simulink model "C28069_LLC_ePWM_V8_230307_PhaeShiftWorking"  (R2022b)
settings: Solver=FixedStepAuto  StartTime=0.0  StopTime=10  RelTol=1e-3  EnableMultiTasking=on
model workspace (MAT data in the model file):
  Comp_DAC = 512
undefined symbols (not defined in the file or in its folder): Down, GPTRIP1SEL, GPTRIP2SEL, PWM_Control, PWM_Gen, PWM_Gen1, SCI_A_Transmit, SCI_A_Transmit_Current_Suffix, SCI_A_Transmit_Duty_Suffix, SCI_A_Transmit_Freq_Suffix, SCI_A_Transmit_OVPFlag_Suffix, SCI_A_Transmit_PFC_Suffix, SCI_A_Transmit_SS_Suffix, SCI_A_Transmit_TBPHS_Suffix, SCI_A_Transmit_VADC_Suffix, SCI_A_Transmit_VAvg_Suffix, SCI_A_Transmit_VBAT_Suffix, SCI_A_Transmit_VBATRef_Suffix, SCI_A_Transmit_Vo_Suffix, TZ1, TZ2, u1, Up
libraries: c2802xlib x92, c280xlib x39, simulink x36, c2000lib x1
(part 17 of 18)

== stateflow chart C28069_LLC_ePWM_V8_230307_PhaeShiftWorking/Softstart @5kHz/GetADC, FaultProtection, SoftStart  @5KHz/SoftStart/If Action Subsystem/SoftStart/Chart1 ==
  note: Under 5KHz, 1 = 0.0002s/cycle
      | 1000 = 0.2s per increment/decrement
  note: [Frequency_Adjusted == Resonant_Frequency]
      | will go here
  note: To initialise the frequency
  (default) -> (junction 47)
  (junction 47) -> (junction 62) [order 2]
  (junction 62) -> (junction 64) : {
      | First_Pass = 1;
      | Soft_Start = 1;
      | Local_counter = 1;
      | SoftStart_OK = 0;
      | }
  (junction 47) -> (junction 48) [order 1] : [PFC_OK]
  (junction 48) -> (junction 49) [order 1] : [First_Pass]
  (junction 48) -> (junction 56) [order 2] : [Soft_Start]
  (junction 56) -> (junction 58) [order 1] : [Local_counter > 400]
      | {
      | Local_counter = 0;
      | }
  (junction 58) -> (junction 74) [order 2]
  (junction 74) -> (junction 81) [order 1] : [[abs(Frequency_Adjusted - Resonant_Frequency)<1]]
  (junction 49) -> (junction 60) : {
      | Frequency_Adjusted = Initial_Frequency;
      | First_Pass = 0;
      | }
  (junction 48) -> (junction 51) [order 3]
  (junction 56) -> (junction 70) [order 2] : {
      | Local_counter = Local_counter +1;
      | }
  (junction 58) -> (junction 68) [order 1] : [Frequency_Adjusted > Resonant_Frequency]
      | {
      | Frequency_Adjusted = Frequency_Adjusted - 0.1;
      | }
  (junction 74) -> (junction 76) [order 2] : [Frequency_Adjusted < Resonant_Frequency]
      |
      | {
      | Frequency_Adjusted = Frequency_Adjusted + 0.1;
      | }
  (junction 81) -> (junction 84) : {
      | SoftStart_OK = 1;
      | Soft_Start = 0;
      | %Frequency_Adjusted = Initial_Frequency;
      | }
  (junction 64) -> (junction 60)
  (junction 60) -> (junction 51)
  (junction 51) -> (junction 70)
  (junction 70) -> (junction 68)
  (junction 68) -> (junction 76)
  (junction 84) -> (junction 76)
  data: SoftStart_OK output; PFC_OK input; Initial_Frequency input; Resonant_Frequency input; Local_counter local =1; Frequency_Adjusted output; First_Pass local =1; Soft_Start local =1

== stateflow chart C28069_LLC_ePWM_V8_230307_PhaeShiftWorking/Softstart @5kHz/GetADC, FaultProtection, SoftStart  @5KHz/SoftStart1/If Action Subsystem/ReservseSoftStart1/Chart1 ==
  note: Under 5KHz, 1 = 0.0002s/cycle
      | 1000 = 0.2s per increment/decrement
  note: [Frequency_Adjusted == Resonant_Frequency]
      | will go here
  note: To initialise the frequency
  note: For increment of 110 (+-5% each DC)
      | Duty_Adjusted @ 660 = 15% Duty
      | '' @ 770 = 10% Duty
      | - - - - - - - - - - - - - - - -
      | 715 + 55 = 15% DutyCycle
      | 660 + 55 (+-2.5%DC) = ~18% DutyCycle = 1us (Minimum required)
  (default) -> (junction 47)
  (junction 47) -> (junction 62) [order 2]
  (junction 62) -> (junction 64) : {
      | First_Pass = 1;
      | Soft_Start = 1;
      | Local_counter = 1;
      | SoftStart_OK = 0;
      | Duty_Adjusted = 100;
      | }
  (junction 47) -> (junction 48) [order 1] : [PFC_OK]
  (junction 48) -> (junction 49) [order 1] : [First_Pass]
  (junction 48) -> (junction 56) [order 2] : [Soft_Start]
  (junction 56) -> (junction 58) [order 1] : [Local_counter > 600]
      | {
      | Local_counter = 0;
      | }
  (junction 58) -> (junction 74) [order 2]
  (junction 74) -> (junction 81) [order 1] : [abs(Frequency_Adjusted - Resonant_Frequency)<1]
  (junction 48) -> (junction 105) [order 4]
  (junction 49) -> (junction 60) : {
      | Frequency_Adjusted = Initial_Frequency;
      | First_Pass = 0;
      | }
  (junction 48) -> (junction 102) [order 3] : [Duty_Adjusted <= 550]
  (junction 56) -> (junction 70) [order 2] : {
      | Local_counter = Local_counter +1;
      | }
  (junction 58) -> (junction 68) [order 1] : [Frequency_Adjusted > Resonant_Frequency]
      | {
      | Frequency_Adjusted = Frequency_Adjusted - 0.1;
      | }
  (junction 74) -> (junction 76) [order 2] : [Frequency_Adjusted < Resonant_Frequency]
      |
      | {
      | Frequency_Adjusted = Frequency_Adjusted + 0.1;
      | }
  (junction 81) -> (junction 84) : {
      | SoftStart_OK = 1;
      | Soft_Start = 0;
      | %%Frequency_Adjusted = Initial_Frequency;
      | }
  (junction 102) -> (junction 105) [order 2] : {
      | Local_counter = Local_counter +1;
      | }
  (junction 105) -> (junction 51)
  (junction 102) -> (junction 108) [order 1] : [Local_counter >600]
      | {
      | Local_counter = 0;
      | }
  (junction 108) -> (junction 51) : {
      | Duty_Adjusted = Duty_Adjusted + 55;
      | }
  (junction 64) -> (junction 60)
  (junction 60) -> (junction 51)
  (junction 51) -> (junction 70)
  (junction 70) -> (junction 68)
  (junction 68) -> (junction 76)
  (junction 84) -> (junction 76)
  data: SoftStart_OK output; Duty_Adjusted output =100; PFC_OK input; Initial_Frequency input; Resonant_Frequency input; Local_counter local =1; Frequency_Adjusted output double; First_Pass local =1; Soft_Start local =1

== stateflow chart C28069_LLC_ePWM_V8_230307_PhaeShiftWorking/Softstart @5kHz/GetADC, FaultProtection, SoftStart  @5KHz/SoftStart1/If Action Subsystem/SoftStart1/Chart ==
  note: Verror = Vbulk_Ref_ADC_adjusted - Vbulk_ADC;
  note: Local variables
      | VbusRefTemp
      | SoftStartCnt
  (default) -> (junction 47)
  (junction 47) -> (junction 50) [order 2]
  (junction 50) -> (junction 52) : {
      | %First_Pass=1;
      | %Soft_Start=1;
      | %SoftStartCnt=1;
      | %Debug=1;
      | }
  (junction 47) -> (junction 5) [order 1] : [PFC_OK]
  (junction 5) -> (junction 7) [order 1] : [First_Pass]
  (junction 5) -> (junction 15) [order 2] : [Soft_Start]
  (junction 15) -> (junction 18) [order 1] : [SoftStartCnt>15]
      | %% 1 count = 0.2ms (5kHz)
      | %% 10 counts = 2ms
  (junction 18) -> (junction 23) [order 2] : %{Debug=Vbulk_Ref_ADC_adjusted;}
  (junction 23) -> (junction 31) : %{Debug=6;}
  (junction 31) -> (junction 55) [order 1] : [abs(VBAT_Ref_adjusted - VBAT_Ref)<0.9]
  (junction 7) -> (junction 10) : {
      | VBAT_Ref_adjusted = VBAT_Value/30;
      | %Vbulk_Ref_ADC_adjusted = Vbulk_Ref_ADC;
      | First_Pass = 0;
      | %Debug=2;
      |
      | }
  (junction 5) -> (junction 38) [order 3] : {
      | SoftStart_OK = 1;
      | %Debug=3;
      | %Vbulk_Ref_ADC_adjusted=Vbulk_Ref_ADC;
      | }
  (junction 15) -> (junction 20) [order 2] : {
      | SoftStartCnt = SoftStartCnt + 1;
      | %Debug=4;
      | }
      | %% incerase the counter first.
  (junction 18) -> (junction 64) [order 1] : [VBAT_Ref_adjusted < VBAT_Ref]
      | {VBAT_Ref_adjusted = VBAT_Ref_adjusted + 0.1;}
      | %% Increase the reference voltage
  (junction 23) -> (junction 26) [commented out] : [VBAT_Ref_adjusted > VBAT_Ref]
      | {VBAT_Ref_adjusted = VBAT_Ref_adjusted - 0.1;
      | }
      | %% Reduce the reference voltage
  (junction 31) -> (junction 33) [order 2] : {
      | Soft_Start=0;
      | SoftStartCnt=0;
      | %Debug=7;
      | VBAT_Ref_adjusted=VBAT_Ref;
      | }
      | %% End soft start
  (junction 55) -> (junction 57) : {
      | Soft_Start=0;
      | SoftStartCnt=0;
      | VBAT_Ref_adjusted=VBAT_Ref;
      | %Debug=8;
      | }
  (junction 64) -> (junction 28) [order 2]
  (junction 64) -> (junction 28) [order 1] : [VBAT_Ref_adjusted < (VBAT_Value/30)]
      | {VBAT_Ref_adjusted = (VBAT_Value/30) ;}
      | %% Increase the reference voltage
  (junction 52) -> (junction 10)
  (junction 10) -> (junction 38)
  (junction 26) -> (junction 28)
  (junction 33) -> (junction 26)
  (junction 57) -> (junction 33)
  (junction 20) -> (junction 38)
  (junction 28) -> (junction 20)
  data: PFC_OK input; VBAT_Value input; VbusRefTemp local =0; SoftStartCnt local =0; VBAT_Ref input double; VBAT_Ref_adjusted output double =0; Vbulk_Ref_ADC_Hard_Value local =0; First_Pass1 local; First_Pass local =1; Soft_Start local =1; SoftStart_OK output

== stateflow chart C28069_LLC_ePWM_V8_230307_PhaeShiftWorking/Softstart @5kHz/GetADC, FaultProtection, SoftStart  @5KHz/SoftStart1/If Action Subsystem/SoftStart1/Chart1 ==
  note: Under 5KHz, 1 = 0.0002s/cycle
      | 1000 = 0.2s per increment/decrement
  note: [Frequency_Adjusted == Resonant_Frequency]
      | will go here
  note: To initialise the frequency
  (default) -> (junction 47)
  (junction 47) -> (junction 62) [order 2]
  (junction 62) -> (junction 64) : {
      | First_Pass = 1;
      | Soft_Start = 1;
      | Local_counter = 1;
      | SoftStart_OK = 0;
      | }
  (junction 47) -> (junction 48) [order 1] : [PFC_OK]
  (junction 48) -> (junction 49) [order 1] : [First_Pass]
  (junction 48) -> (junction 56) [order 2] : [Soft_Start]
  (junction 56) -> (junction 58) [order 1] : [Local_counter > 400]
      | {
      | Local_counter = 0;
      | }
  (junction 58) -> (junction 74) [order 2]
  (junction 74) -> (junction 81) [order 1] : [[abs(Frequency_Adjusted - Resonant_Frequency)<1]]
  (junction 49) -> (junction 60) : {
      | Frequency_Adjusted = Initial_Frequency;
      | First_Pass = 0;
      | }
  (junction 48) -> (junction 51) [order 3]
  (junction 56) -> (junction 70) [order 2] : {
      | Local_counter = Local_counter +1;
      | }
  (junction 58) -> (junction 68) [order 1] : [Frequency_Adjusted > Resonant_Frequency]
      | {
      | Frequency_Adjusted = Frequency_Adjusted - 0.1;
      | }
  (junction 74) -> (junction 76) [order 2] : [Frequency_Adjusted < Resonant_Frequency]
      |
      | {
      | Frequency_Adjusted = Frequency_Adjusted + 0.1;
      | }
  (junction 81) -> (junction 84) : {
      | SoftStart_OK = 1;
      | Soft_Start = 0;
      | %Frequency_Adjusted = Initial_Frequency;
      | }
  (junction 64) -> (junction 60)
  (junction 60) -> (junction 51)
  (junction 51) -> (junction 70)
  (junction 70) -> (junction 68)
  (junction 68) -> (junction 76)
  (junction 84) -> (junction 76)
  data: SoftStart_OK output; PFC_OK input; Initial_Frequency input; Resonant_Frequency input; Local_counter local =1; Frequency_Adjusted output; First_Pass local =1; Soft_Start local =1

== stateflow chart C28069_LLC_ePWM_V8_230307_PhaeShiftWorking/Softstart @5kHz/GetADC, FaultProtection, SoftStart  @5KHz/SoftStart1/ReservseSoftStart/Chart1 ==
  note: Under 5KHz, 1 = 0.0002s/cycle
      | 1000 = 0.2s per increment/decrement
  note: [Frequency_Adjusted == Resonant_Frequency]
      | will go here
  note: To initialise the frequency
  note: For increment of 110 (+-5% each DC)
      | Duty_Adjusted @ 660 = 15% Duty
      | '' @ 770 = 10% Duty
      | - - - - - - - - - - - - - - - -
      | 715 + 55 = 15% DutyCycle
      | 660 + 55 (+-2.5%DC) = ~18% DutyCycle = 1us (Minimum required)
  (default) -> (junction 47)
  (junction 47) -> (junction 62) [order 2]
  (junction 62) -> (junction 64) : {
      | First_Pass = 1;
      | Soft_Start = 1;
      | Local_counter = 1;
      | SoftStart_OK = 0;
      | Duty_Adjusted = 100;
      | }
  (junction 47) -> (junction 48) [order 1] : [PFC_OK]
  (junction 48) -> (junction 49) [order 1] : [First_Pass]
  (junction 48) -> (junction 56) [order 2] : [Soft_Start]
  (junction 56) -> (junction 58) [order 1] : [Local_counter > 600]
      | {
      | Local_counter = 0;
      | }
  (junction 58) -> (junction 74) [order 2]
  (junction 74) -> (junction 81) [order 1] : [abs(Frequency_Adjusted - Resonant_Frequency)<1]
  (junction 48) -> (junction 105) [order 4]
  (junction 49) -> (junction 60) : {
      | Frequency_Adjusted = Initial_Frequency;
      | First_Pass = 0;
      | }
  (junction 48) -> (junction 102) [order 3] : [Duty_Adjusted <= 550]
  (junction 56) -> (junction 70) [order 2] : {
      | Local_counter = Local_counter +1;
      | }
  (junction 58) -> (junction 68) [order 1] : [Frequency_Adjusted > Resonant_Frequency]
      | {
      | Frequency_Adjusted = Frequency_Adjusted - 0.1;
      | }
  (junction 74) -> (junction 76) [order 2] : [Frequency_Adjusted < Resonant_Frequency]
      |
      | {
      | Frequency_Adjusted = Frequency_Adjusted + 0.1;
      | }
  (junction 81) -> (junction 84) : {
      | SoftStart_OK = 1;
      | Soft_Start = 0;
      | %%Frequency_Adjusted = Initial_Frequency;
      | }
  (junction 102) -> (junction 105) [order 2] : {
      | Local_counter = Local_counter +1;
      | }
  (junction 105) -> (junction 51)
  (junction 102) -> (junction 108) [order 1] : [Local_counter >600]
      | {
      | Local_counter = 0;
      | }
  (junction 108) -> (junction 51) : {
      | Duty_Adjusted = Duty_Adjusted + 55;
      | }
  (junction 64) -> (junction 60)
  (junction 60) -> (junction 51)
  (junction 51) -> (junction 70)
  (junction 70) -> (junction 68)
  (junction 68) -> (junction 76)
  (junction 84) -> (junction 76)
  data: SoftStart_OK output; Duty_Adjusted output =100; PFC_OK input; Initial_Frequency input; Resonant_Frequency input; Local_counter local =1; Frequency_Adjusted output double; First_Pass local =1; Soft_Start local =1

== stateflow chart C28069_LLC_ePWM_V8_230307_PhaeShiftWorking/GetADC, FaultProtection, SoftStart  @5KHz/Counter with reset Min output = 1 Max output = Counter reset value ==
  (default) -> (junction 1)
  (junction 1) -> (junction 17) [order 2]
  (junction 1) -> (junction 3) [order 1]
  (junction 17) -> (junction 19) : [(Counter==Number_of_counts) & Latch_switch]
      | {Counter=Number_of_counts;}
  (junction 1) -> (junction 7) [order 3] : {Counter = Counter + 1;}
  (junction 3) -> (junction 5) : [(Counter==Number_of_counts+1) & (~Latch_switch)]
      | {Counter=1;}
  (junction 19) -> (junction 7)
  (junction 5) -> (junction 7)
  data: Number_of_counts input; Counter output double =0; Latch_switch input

== stateflow chart C28069_LLC_ePWM_V8_230307_PhaeShiftWorking/Softstart @5kHz/GetADC, FaultProtection, SoftStart  @5KHz/SoftStart1/SoftStart/Chart ==
  note: Verror = Vbulk_Ref_ADC_adjusted - Vbulk_ADC;
  note: Local variables
      | VbusRefTemp
      | SoftStartCnt
  (default) -> (junction 47)
  (junction 47) -> (junction 50) [order 2]
  (junction 50) -> (junction 52) : {
      | First_Pass=1;
      | Soft_Start=1;
      | SoftStartCnt=1;
      | %Debug=1;
      | }
  (junction 47) -> (junction 5) [order 1] : [PFC_OK]
  (junction 5) -> (junction 7) [order 1] : [First_Pass]
  (junction 5) -> (junction 15) [order 2] : [Soft_Start]
  (junction 15) -> (junction 18) [order 1] : [SoftStartCnt>100]
      | %% At every 5 cycles (total 1ms),
  (junction 18) -> (junction 23) [order 2] : %{Debug=Vbulk_Ref_ADC_adjusted;}
  (junction 23) -> (junction 31) [order 2] : %{Debug=6;}
  (junction 31) -> (junction 55) [order 1] : [abs(VBAT_Ref_adjusted - VBAT_Ref)<1]
  (junction 7) -> (junction 10) : {
      | VBAT_Ref_adjusted = VBAT_Value;
      | %Vbulk_Ref_ADC_adjusted = Vbulk_Ref_ADC;
      | First_Pass = 0;
      | %Debug=2;
      |
      | }
  (junction 5) -> (junction 38) [order 3] : {
      | %Debug=3;
      | %Vbulk_Ref_ADC_adjusted=Vbulk_Ref_ADC;
      | }
  (junction 15) -> (junction 20) [order 2] : {
      | SoftStartCnt = SoftStartCnt + 1;
      | %Debug=4;
      | }
      | %% incerase the counter first.
  (junction 18) -> (junction 64) [order 1] : [VBAT_Ref_adjusted < VBAT_Ref]
      | {VBAT_Ref_adjusted = VBAT_Ref_adjusted + 0.1;}
      | %% Increase the reference voltage
  (junction 23) -> (junction 26) [order 1] : [VBAT_Ref_adjusted > VBAT_Ref]
      | {VBAT_Ref_adjusted = VBAT_Ref_adjusted - 0.1;
      | }
      | %% Reduce the reference voltage
  (junction 31) -> (junction 33) [order 2] : {
      | Soft_Start=0;
      | SoftStartCnt=0;
      | %Debug=7;
      | }
      | %% End soft start
  (junction 55) -> (junction 57) : {
      | Soft_Start=0;
      | SoftStartCnt=0;
      | VBAT_Ref_adjusted=VBAT_Ref;
      | %Debug=8;
      | }
  (junction 64) -> (junction 28) [order 2]
  (junction 64) -> (junction 28) [order 1] : [VBAT_Ref_adjusted < VBAT_Value]
      | {VBAT_Ref_adjusted = VBAT_Value ;}
      | %% Increase the reference voltage
  (junction 52) -> (junction 10)
  (junction 10) -> (junction 38)
  (junction 26) -> (junction 28)
  (junction 33) -> (junction 26)
  (junction 57) -> (junction 33)
  (junction 20) -> (junction 38)
  (junction 28) -> (junction 20)
  data: PFC_OK input; VBAT_Value input; VbusRefTemp local =0; SoftStartCnt local =0; VBAT_Ref input double; VBAT_Ref_adjusted output double =0; Vbulk_Ref_ADC_Hard_Value local =0; First_Pass1 local; First_Pass local =1; Soft_Start local =1

== stateflow chart C28069_LLC_ePWM_V8_230307_PhaeShiftWorking/Softstart @5kHz/GetADC, FaultProtection, SoftStart  @5KHz/SoftStart1/SoftStart/Chart1 ==
  note: Under 5KHz, 1 = 0.0002s/cycle
      | 1000 = 0.2s per increment/decrement
  note: [Frequency_Adjusted == Resonant_Frequency]
      | will go here
  note: To initialise the frequency
  (default) -> (junction 47)
  (junction 47) -> (junction 62) [order 2]
  (junction 62) -> (junction 64) : {
      | First_Pass = 1;
      | Soft_Start = 1;
      | Local_counter = 1;
      | SoftStart_OK = 0;
      | }
  (junction 47) -> (junction 48) [order 1] : [PFC_OK]
  (junction 48) -> (junction 49) [order 1] : [First_Pass]
  (junction 48) -> (junction 56) [order 2] : [Soft_Start]
  (junction 56) -> (junction 58) [order 1] : [Local_counter > 400]
      | {
      | Local_counter = 0;
      | }
  (junction 58) -> (junction 74) [order 2]
  (junction 74) -> (junction 81) [order 1] : [[abs(Frequency_Adjusted - Resonant_Frequency)<1]]
  (junction 49) -> (junction 60) : {
      | Frequency_Adjusted = Initial_Frequency;
      | First_Pass = 0;
      | }
  (junction 48) -> (junction 51) [order 3]
  (junction 56) -> (junction 70) [order 2] : {
      | Local_counter = Local_counter +1;
      | }
  (junction 58) -> (junction 68) [order 1] : [Frequency_Adjusted > Resonant_Frequency]
      | {
      | Frequency_Adjusted = Frequency_Adjusted - 0.1;
      | }
  (junction 74) -> (junction 76) [order 2] : [Frequency_Adjusted < Resonant_Frequency]
      |
      | {
      | Frequency_Adjusted = Frequency_Adjusted + 0.1;
      | }
  (junction 81) -> (junction 84) : {
      | SoftStart_OK = 1;
      | Soft_Start = 0;
      | %Frequency_Adjusted = Initial_Frequency;
      | }
  (junction 64) -> (junction 60)
  (junction 60) -> (junction 51)
  (junction 51) -> (junction 70)
  (junction 70) -> (junction 68)
  (junction 68) -> (junction 76)
  (junction 84) -> (junction 76)
  data: SoftStart_OK output; PFC_OK input; Initial_Frequency input; Resonant_Frequency input; Local_counter local =1; Frequency_Adjusted output; First_Pass local =1; Soft_Start local =1

== stateflow chart C28069_LLC_ePWM_V8_230307_PhaeShiftWorking/Softstart @5kHz/GetADC, FaultProtection, SoftStart  @5KHz/UpdatePWM/Close Loop Regulation/If Action Subsystem/Chart ==
  note: Note
      | Voltage drop = Freq increase
  note: When Actual voltage is higher
  note: When Actual voltage is lower
  (default) -> (junction 1)
  (junction 1) -> (junction 16) [order 1] : [input_u>0]{output_y=prev_freq-0.01;}
  (junction 1) -> (junction 17) [order 2] : {output_y=prev_freq+0.01;}
  (junction 16) -> (junction 19) [order 1] : [output_y<100]{output_y=100;}
  (junction 17) -> (junction 19) [order 1] : [output_y>180]{output_y=180;}
  (junction 17) -> (junction 32) [order 2]
  (junction 16) -> (junction 34) [order 2]
  (junction 32) -> (junction 19)
  (junction 34) -> (junction 19)
  (junction 19) -> (junction 22)
  data: output_y output double; input_u input double; prev_freq input double

== stateflow chart C28069_LLC_ePWM_V8_230307_PhaeShiftWorking/CloseLoop & Update @ ADCINT, 50kHz/Close Loop Regulation1/If Action Subsystem/Chart1 ==
  note: [output_freq>180]
      | {
      | output_freq=180;
      | output_deadband =  output_deadband + 1;
      | }
  (default) -> (junction 221)
  (junction 221) -> (junction 223) : {
      | %%y(k) = b0*e(k) + b1*e(k-1) - a1*y(k-1)
      | output_freq = (b0*error) + (b1*error_z1) - (a1*output_z1);
      | }
  (junction 223) -> (junction 239) [order 2] : [output_freq<0.65]
  (junction 223) -> (junction 243) [order 3]
  (junction 239) -> (junction 241) : {output_freq=0.65;}
  (junction 223) -> (junction 225) [order 1] : [output_freq>1.5]
  (junction 243) -> (junction 245)
  (junction 225) -> (junction 237) : {output_freq=1.5;}
  (junction 241) -> (junction 237)
  (junction 245) -> (junction 237)
  (junction 237) -> (junction 233) : {
      | output_z1 = output_freq;
      | error_z1 = error;
      | }
  data: output_freq output double =0; error input double; prev_freq input double; b0 input; b1 input; a1 input; error_z1 local =0; output_z1 local =0

== matlab function C28069_LLC_ePWM_V8_230307_PhaeShiftWorking/UART Reporting @ 1Hz/SCI_A_Transmit_function2/MATLAB Function ==
  data: Main_number input; Digit_5 output; Divider input; Digit_4 output; Digit_3 output; Digit_2 output; Digit_1 output
function [Digit_5,Digit_4,Digit_3,Digit_2,Digit_1]  = fcn(Main_number,Divider)

R_Digit_5 = rem(Main_number,Divider);
Q_Digit_5 = (Main_number-R_Digit_5)/Divider;
Digit_5 = uint8(Q_Digit_5);
%Digit_5 done

R_Digit_4 = rem(R_Digit_5,Divider/10);
Q_Digit_4 = (R_Digit_5-R_Digit_4)/(Divider/10);
Digit_4 = uint8(Q_Digit_4);
%Digit_4 done

R_Digit_3 = rem(R_Digit_4,Divider/100);
Q_Digit_3 = (R_Digit_4-R_Digit_3)/(Divider/100);
Digit_3 = uint8(Q_Digit_3);
%Digit_3 done

R_Digit_2 = rem(R_Digit_3,Divider/1000);
Q_Digit_2 = (R_Digit_3-R_Digit_2)/(Divider/1000);
Digit_2 = uint8(Q_Digit_2);
%Digit_2 done

R_Digit_1 = rem(R_Digit_2,Divider/10000);
Q_Digit_1 = (R_Digit_2-R_Digit_1)/(Divider/10000);
Digit_1 = uint8(Q_Digit_1);
%Digit_1 done
end

== stateflow chart C28069_LLC_ePWM_V8_230307_PhaeShiftWorking/CloseLoop & Update @ ADCINT, 50kHz/Close Loop Regulation1/If Action Subsystem/Chart2 ==
  note: Note
      | Voltage drop = Freq increase
  note: When Actual voltage is higher
  note: When Actual voltage is lower
  note: Note
      | Voltage drop = Freq increase
  note: When Actual voltage is lower
  note: When Actual voltage is higher
  note: If <25V & <47% & freq is 180K
  note: Minor delay of 1KHz,
      | 1 count = 1ms
      | 100 = 100ms delay
  note: Increase Duty
  note: Reduce Duty
  (default) -> (junction 1)
  (junction 17) -> (junction 145) [order 2]
  (junction 1) -> (junction 17) [order 2] : {output_freq=prev_freq+0.05;}
  (junction 1) -> (junction 157) [order 1] : [error>0]
  (junction 157) -> (junction 184) [order 2]
  (junction 184) -> (junction 164) [order 2]
  (junction 145) -> (junction 152)
  (junction 17) -> (junction 141) [order 1] : [output_freq>180]
      | {
      | output_freq=180;
      | output_deadband =  output_deadband + 1;
      | }
  (junction 157) -> (junction 181) [order 1] : [output_deadband>1]
      | {output_deadband = output_deadband - 1;}
  (junction 184) -> (junction 187) [order 1] : [output_freq==0]
      | {output_freq=180;}
  (junction 164) -> (junction 166) : {output_freq=output_freq-0.05;}
  (junction 166) -> (junction 177) [order 2]
  (junction 166) -> (junction 171) [order 1] : [output_freq<100]{output_freq=100;}
  (junction 177) -> (junction 175)
  (junction 141) -> (junction 152) [order 2]
  (junction 152) -> (junction 147)
  (junction 141) -> (junction 143) [order 1] : [output_deadband > 660]
      | {
      | output_deadband = 660;
      | output_freq=0;
      | }
  (junction 147) -> (junction 143)
  (junction 143) -> (junction 181)
  (junction 187) -> (junction 181)
  (junction 171) -> (junction 187)
  (junction 175) -> (junction 171)
  (default) -> (junction 94) [commented out]
  (junction 94) -> (junction 101) [commented out] : {output_freq=prev_freq+0.05;}
  (junction 94) -> (junction 89) [commented out] : [error>0]{output_freq=prev_freq-0.05;}
  (junction 101) -> (junction 98) [commented out] : [output_freq>180]
      | {
      | output_freq=180;
      | %limit_cap = limit_cap + 1;
      | }
  (junction 94) -> (junction 96) [commented out] : [input_u> 0 & duty_output > 56 & prev_freq ==180]
  (junction 89) -> (junction 108) [commented out]
  (junction 101) -> (junction 103) [commented out]
  (junction 89) -> (junction 108) [commented out] : [output_freq<100]{output_freq=100;}
  (junction 98) -> (junction 105) [commented out] : [input_u<0]
  (junction 98) -> (junction 97) [commented out]
  (junction 96) -> (junction 132) [commented out] : {
      | duty_output = duty_output - 55;
      | }
  (junction 105) -> (junction 113) [commented out] : %Need to send CMPA 0 not duty
      | %{duty_output = 0;}
  (junction 105) -> (junction 99) [commented out] : [duty_output <= 660]
  (junction 97) -> (junction 134) [commented out] : %{limit_cap = 0;}
  (junction 99) -> (junction 90) [commented out]
  (junction 99) -> (junction 100) [commented out] : [Local_counter > 600]
      | {
      | Local_counter = 0;
      | }
  (junction 90) -> (junction 113) [commented out] : {Local_counter = Local_counter + 1;}
  (junction 100) -> (junction 117) [commented out] : {
      | duty_output = duty_output + 55;
      | }
  (junction 103) -> (junction 107) [commented out]
  (junction 107) -> (junction 113) [commented out]
  (junction 113) -> (junction 117) [commented out]
  (junction 134) -> (junction 117) [commented out]
  (junction 132) -> (junction 134) [commented out]
  (junction 108) -> (junction 132) [commented out]
  (junction 117) -> (junction 110) [commented out]
  data: output_freq output double; error input double; prev_freq input double; limit_cap local double =0; Local_counter local =0; output_deadband output

== stateflow chart C28069_LLC_ePWM_V8_230307_PhaeShiftWorking/CloseLoop & Update @ ADCINT, 50kHz/Close Loop Regulation1/If Action Subsystem/Chart3 ==
  note: [output_freq>180]
      | {
      | output_freq=180;
      | output_deadband =  output_deadband + 1;
      | }
  (default) -> (junction 221)
  (junction 221) -> (junction 223) : {
      | %%y(k) = b0*e(k) + b1*e(k-1) - a1*y(k-1)
      | output_freq = (b0*error) + (b1*error_z1) - (a1*output_z1);
      | }
  (junction 223) -> (junction 239) [order 2] : [output_freq<0.65]
  (junction 223) -> (junction 243) [order 3]
  (junction 239) -> (junction 241) : {output_freq=0.65;}
  (junction 223) -> (junction 225) [order 1] : [output_freq>1.5]
  (junction 243) -> (junction 245)
  (junction 225) -> (junction 237) : {output_freq=1.5;}
  (junction 241) -> (junction 237)
  (junction 245) -> (junction 237)
  (junction 237) -> (junction 233) : {
      | output_z1 = output_freq;
      | error_z1 = error;
      | }
  data: output_freq output double =0; error input double; prev_freq input double; b0 input; b1 input; a1 input; error_z1 local =0; output_z1 local =0

== stateflow chart C28069_LLC_ePWM_V8_230307_PhaeShiftWorking/GetADC, FaultProtection, SoftStart  @5KHz/UpdatePWM1/Close Loop Regulation/If Action Subsystem/Chart1 ==
  note: [output_freq>180]
      | {
      | output_freq=180;
      | output_deadband =  output_deadband + 1;
      | }
  (default) -> (junction 221)
  (junction 221) -> (junction 223) : {
      | %%y(k) = b0*e(k) + b1*e(k-1) - a1*y(k-1)
      | output_freq = (b0*error) + (b1*error_z1) - (a1*output_z1);
      | }
  (junction 223) -> (junction 239) [order 2] : [output_freq<0.9]
  (junction 223) -> (junction 243) [order 3]
  (junction 239) -> (junction 241) : {output_freq=0.9;}
  (junction 223) -> (junction 225) [order 1] : [output_freq>1.5]
  (junction 243) -> (junction 245)
  (junction 225) -> (junction 237) : {output_freq=1.5;}
  (junction 241) -> (junction 237)
  (junction 245) -> (junction 237)
  (junction 237) -> (junction 233) : {
      | output_z1 = output_freq;
      | error_z1 = error;
      | }
  data: output_freq output double =0; error input double; prev_freq input double; b0 input; b1 input; a1 input; error_z1 local =0; output_z1 local =0

== stateflow chart C28069_LLC_ePWM_V8_230307_PhaeShiftWorking/CloseLoop & Update @ ADCINT, 50kHz/Close Loop Regulation1/If Action Subsystem/Chart4 ==
  note: lower limit cap
  note: upper limit cap
  note: reduce duty cycle
  note: increase duty cycle
  note: If dutycycle hit certain %,
      | we set pwm to 0
  note: set to upper limit
      | if pwm = 0
  (default) -> (junction 221)
  (junction 221) -> (junction 223) : {
      | %%y(k) = b0*e(k) + b1*e(k-1) - a1*y(k-1)
      | output_freq = (b0*error) + (b1*error_z1) - (a1*output_z1);
      | }
  (junction 223) -> (junction 239) [order 2] : [output_freq<0.65]
  (junction 223) -> (junction 243) [order 3]
  (junction 243) -> (junction 267) [order 2]
  (junction 267) -> (junction 272) [order 2]
  (junction 267) -> (junction 273) [order 1] : [output_freq==0]
      | {output_freq=1.5;}
  (junction 239) -> (junction 241) : {output_freq=0.65;}
  (junction 223) -> (junction 225) [order 1] : [output_freq>1.5]
  (junction 243) -> (junction 245) [order 1] : [output_deadband>1]
      | {output_deadband = output_deadband - 1;}
  (junction 272) -> (junction 275)
  (junction 225) -> (junction 249) : {
      | output_freq=1.5;
      | output_deadband = output_deadband +1;
      | }
  (junction 249) -> (junction 257) [order 2]
  (junction 257) -> (junction 250)
  (junction 249) -> (junction 251) [order 1] : [output_deadband > 660]
      | {
      | output_deadband = 660;
      | output_freq=0;
      | }
  (junction 250) -> (junction 251)
  (junction 251) -> (junction 237)
  (junction 275) -> (junction 273)
  (junction 273) -> (junction 245)
  (junction 241) -> (junction 237)
  (junction 245) -> (junction 237)
  (junction 237) -> (junction 233) : {
      | output_z1 = output_freq;
      | error_z1 = error;
      | }
  data: output_freq output double =0; error input double; prev_freq input double; b0 input; b1 input; a1 input; error_z1 local =0; output_z1 local =0; output_deadband output

== stateflow chart C28069_LLC_ePWM_V8_230307_PhaeShiftWorking/CloseLoop & Update @ ADCINT, 50kHz/Close Loop Regulation1/If Action Subsystem/DefaultWorking ==
  note: Note
      | Voltage drop = Freq increase
  note: When Actual voltage is higher
  note: When Actual voltage is lower
  (default) -> (junction 1)
  (junction 1) -> (junction 17) [order 2] : {output_y=prev_freq+0.01;}
  (junction 1) -> (junction 16) [order 1] : [input_u>0]{output_y=prev_freq-0.01;}
  (junction 16) -> (junction 46) [order 1] : [output_y<100]{output_y=100;}
  (junction 17) -> (junction 48) [order 1] : [output_y>180]
      | {
      | output_y=180;
      | limit_cap = limit_cap + 1;
      | }
  (junction 17) -> (junction 32) [order 2]
  (junction 16) -> (junction 34) [order 2]
  (junction 32) -> (junction 48)
  (junction 48) -> (junction 65)
  (junction 65) -> (junction 19)
  (junction 71) -> (junction 19)
  (junction 59) -> (junction 71)
  (junction 46) -> (junction 59)
  (junction 34) -> (junction 46)
  (junction 19) -> (junction 22)
  data: output_y output double; input_u input double; prev_freq input double; limit_cap local double =0; Local_Counter local =0

== stateflow chart C28069_LLC_ePWM_V8_230307_PhaeShiftWorking/CloseLoop & Update @ ADCINT, 50kHz/Close Loop Regulation1/If Action Subsystem/Working & Added Delay Counter ==
  note: Note
      | Voltage drop = Freq increase
  note: When Actual voltage is higher
  note: When Actual voltage is lower
  note: Note
      | Voltage drop = Freq increase
  note: When Actual voltage is lower
  note: When Actual voltage is higher
  note: If <25V & <47% & freq is 180K
  note: Minor delay of 1KHz,
      | 1 count = 1ms
      | 100 = 100ms delay
  note: Increase Duty
  note: Reduce Duty
  (default) -> (junction 1)
  (junction 17) -> (junction 145) [order 2]
  (junction 1) -> (junction 17) [order 2] : {output_freq=prev_freq+0.05;}
  (junction 1) -> (junction 157) [order 1] : [error>0]
  (junction 157) -> (junction 184) [order 2]
  (junction 184) -> (junction 164) [order 2]
  (junction 145) -> (junction 152)
  (junction 17) -> (junction 201) [order 1] : [output_freq>180]
      | {
      | output_freq=180;
      | %output_deadband =  output_deadband + 1;
      | }
  (junction 157) -> (junction 209) [order 1] : [output_deadband>1]
      | %{output_deadband = output_deadband - 1;}
  (junction 184) -> (junction 187) [order 1] : [output_freq==0]
      | {output_freq=180;}
  (junction 164) -> (junction 166) : {output_freq=output_freq-0.05;}
  (junction 166) -> (junction 177) [order 2]
  (junction 166) -> (junction 171) [order 1] : [output_freq<100]{output_freq=100;}
  (junction 177) -> (junction 175)
  (junction 201) -> (junction 204) [order 2] : {Local_counter = Local_counter + 1;}
  (junction 201) -> (junction 206) [order 1] : [Local_counter > 10]
      | {Local_counter = 0;}
  (junction 209) -> (junction 211) [order 1] : [Local_counter > 10]
      | {Local_counter = 0;}
  (junction 209) -> (junction 212) [order 2] : {Local_counter = Local_counter + 1;}
  (junction 204) -> (junction 141)
  (junction 206) -> (junction 141) : {output_deadband =  output_deadband + 1;}
  (junction 212) -> (junction 181)
  (junction 211) -> (junction 181) : {output_deadband = output_deadband - 1;}
  (junction 141) -> (junction 152) [order 2]
  (junction 152) -> (junction 147)
  (junction 141) -> (junction 143) [order 1] : [output_deadband > 660]
      | {
      | output_deadband = 660;
      | output_freq=0;
      | }
  (junction 147) -> (junction 143)
  (junction 143) -> (junction 181)
  (junction 187) -> (junction 181)
  (junction 171) -> (junction 187)
  (junction 175) -> (junction 171)
  (default) -> (junction 94) [commented out]
  (junction 94) -> (junction 101) [commented out] : {output_freq=prev_freq+0.05;}
  (junction 94) -> (junction 89) [commented out] : [error>0]{output_freq=prev_freq-0.05;}
  (junction 101) -> (junction 98) [commented out] : [output_freq>180]
      | {
      | output_freq=180;
      | %limit_cap = limit_cap + 1;
      | }
  (junction 94) -> (junction 96) [commented out] : [input_u> 0 & duty_output > 56 & prev_freq ==180]
  (junction 89) -> (junction 108) [commented out]
  (junction 101) -> (junction 103) [commented out]
  (junction 89) -> (junction 108) [commented out] : [output_freq<100]{output_freq=100;}
  (junction 98) -> (junction 105) [commented out] : [input_u<0]
  (junction 98) -> (junction 97) [commented out]
  (junction 96) -> (junction 132) [commented out] : {
      | duty_output = duty_output - 55;
      | }
  (junction 105) -> (junction 113) [commented out] : %Need to send CMPA 0 not duty
      | %{duty_output = 0;}
  (junction 105) -> (junction 99) [commented out] : [duty_output <= 660]
  (junction 97) -> (junction 134) [commented out] : %{limit_cap = 0;}
  (junction 99) -> (junction 90) [commented out]
  (junction 99) -> (junction 100) [commented out] : [Local_counter > 600]
      | {
      | Local_counter = 0;
      | }
  (junction 90) -> (junction 113) [commented out] : {Local_counter = Local_counter + 1;}
  (junction 100) -> (junction 117) [commented out] : {
      | duty_output = duty_output + 55;
      | }
  (junction 103) -> (junction 107) [commented out]
  (junction 107) -> (junction 113) [commented out]
  (junction 113) -> (junction 117) [commented out]
  (junction 134) -> (junction 117) [commented out]
  (junction 132) -> (junction 134) [commented out]
  (junction 108) -> (junction 132) [commented out]
  (junction 117) -> (junction 110) [commented out]
  data: output_freq output double; error input double; prev_freq input double; limit_cap local double =0; Local_counter local =0; output_deadband output

== stateflow chart C28069_LLC_ePWM_V8_230307_PhaeShiftWorking/CloseLoop & Update @ ADCINT, 50kHz/Get AVG1/Chart1 ==
  (default) -> (junction 1) : {
      | output_y = b0*input_u + b1*input_z1 - a1*output_z1;
      | input_z1 = input_u;
      | output_z1 = output_y;
      | }
  data: input_z1 local =0; output_z1 local =0; output_y output; input_u input; b0 input; b1 input; a1 input

== stateflow chart C28069_LLC_ePWM_V8_230307_PhaeShiftWorking/CloseLoop & Update @ ADCINT, 50kHz/Get AVG1/Chart2 ==
  (default) -> (junction 1) : {
      | output_y = b0*input_u + b1*input_z1 - a1*output_z1;
      | input_z1 = input_u;
      | output_z1 = output_y;
      | }
  data: input_z1 local =0; output_z1 local =0; output_y output; input_u input; b0 input; b1 input; a1 input

== stateflow chart C28069_LLC_ePWM_V8_230307_PhaeShiftWorking/GetADC Measurement @50kHz/Chart1 ==
  (default) -> (junction 1) : {
      | output_y = b0*input_u + b1*input_z1 - a1*output_z1;
      | input_z1 = input_u;
      | output_z1 = output_y;
      | }
  data: input_z1 local =0; output_z1 local =0; output_y output; input_u input; b0 input; b1 input; a1 input

== stateflow chart C28069_LLC_ePWM_V8_230307_PhaeShiftWorking/CloseLoop & Update @ ADCINT, 50kHz/Close Loop Regulation2/If Action Subsystem/Chart2 ==
  note: Note
      | Voltage drop = Freq increase
  note: When Actual voltage is higher
  note: When Actual voltage is lower
  note: Note
      | Voltage drop = Freq increase
  note: When Actual voltage is lower
  note: When Actual voltage is higher
  note: If <25V & <47% & freq is 180K
  note: Minor delay of 1KHz,
      | 1 count = 1ms
      | 100 = 100ms delay
  note: Increase Duty
  note: Reduce Duty
  (default) -> (junction 1)
  (junction 17) -> (junction 145) [order 2]
  (junction 1) -> (junction 17) [order 2] : {output_freq=prev_freq+0.05;}
  (junction 1) -> (junction 157) [order 1] : [error>0]
  (junction 157) -> (junction 184) [order 2]
  (junction 184) -> (junction 164) [order 2]
  (junction 145) -> (junction 152)
  (junction 17) -> (junction 141) [order 1] : [output_freq>180]
      | {
      | output_freq=180;
      | output_deadband =  output_deadband + 1;
      | }
  (junction 157) -> (junction 181) [order 1] : [output_deadband>1]
      | {output_deadband = output_deadband - 1;}
  (junction 184) -> (junction 187) [order 1] : [output_freq==0]
      | {output_freq=180;}
  (junction 164) -> (junction 166) : {output_freq=output_freq-0.05;}
  (junction 166) -> (junction 177) [order 2]
  (junction 166) -> (junction 171) [order 1] : [output_freq<100]{output_freq=100;}
  (junction 177) -> (junction 175)
  (junction 141) -> (junction 152) [order 2]
  (junction 152) -> (junction 147)
  (junction 141) -> (junction 143) [order 1] : [output_deadband > 660]
      | {
      | output_deadband = 660;
      | output_freq=0;
      | }
  (junction 147) -> (junction 143)
  (junction 143) -> (junction 181)
  (junction 187) -> (junction 181)
  (junction 171) -> (junction 187)
  (junction 175) -> (junction 171)
  (default) -> (junction 94) [commented out]
  (junction 94) -> (junction 101) [commented out] : {output_freq=prev_freq+0.05;}
  (junction 94) -> (junction 89) [commented out] : [error>0]{output_freq=prev_freq-0.05;}
  (junction 101) -> (junction 98) [commented out] : [output_freq>180]
      | {
      | output_freq=180;
      | %limit_cap = limit_cap + 1;
      | }
  (junction 94) -> (junction 96) [commented out] : [input_u> 0 & duty_output > 56 & prev_freq ==180]
  (junction 89) -> (junction 108) [commented out]
  (junction 101) -> (junction 103) [commented out]
  (junction 89) -> (junction 108) [commented out] : [output_freq<100]{output_freq=100;}
  (junction 98) -> (junction 105) [commented out] : [input_u<0]
  (junction 98) -> (junction 97) [commented out]
  (junction 96) -> (junction 132) [commented out] : {
      | duty_output = duty_output - 55;
      | }
  (junction 105) -> (junction 113) [commented out] : %Need to send CMPA 0 not duty
      | %{duty_output = 0;}
  (junction 105) -> (junction 99) [commented out] : [duty_output <= 660]
  (junction 97) -> (junction 134) [commented out] : %{limit_cap = 0;}
  (junction 99) -> (junction 90) [commented out]
  (junction 99) -> (junction 100) [commented out] : [Local_counter > 600]
      | {
      | Local_counter = 0;
      | }
  (junction 90) -> (junction 113) [commented out] : {Local_counter = Local_counter + 1;}
  (junction 100) -> (junction 117) [commented out] : {
      | duty_output = duty_output + 55;
      | }
  (junction 103) -> (junction 107) [commented out]
  (junction 107) -> (junction 113) [commented out]
  (junction 113) -> (junction 117) [commented out]
  (junction 134) -> (junction 117) [commented out]
  (junction 132) -> (junction 134) [commented out]
  (junction 108) -> (junction 132) [commented out]
  (junction 117) -> (junction 110) [commented out]
  data: output_freq output double; error input double; prev_freq input double; limit_cap local double =0; Local_counter local =0; output_deadband output

== matlab function C28069_LLC_ePWM_V8_230307_PhaeShiftWorking/UART Reporting @ 1Hz/SCI_A_Transmit_function9/MATLAB Function ==
  data: Main_number input; Digit_5 output; Divider input; Digit_4 output; Digit_3 output; Digit_2 output; Digit_1 output
function [Digit_5,Digit_4,Digit_3,Digit_2,Digit_1]  = fcn(Main_number,Divider)

R_Digit_5 = rem(Main_number,Divider);
Q_Digit_5 = (Main_number-R_Digit_5)/Divider;
Digit_5 = uint8(Q_Digit_5);
%Digit_5 done

R_Digit_4 = rem(R_Digit_5,Divider/10);
Q_Digit_4 = (R_Digit_5-R_Digit_4)/(Divider/10);
Digit_4 = uint8(Q_Digit_4);
%Digit_4 done

R_Digit_3 = rem(R_Digit_4,Divider/100);
Q_Digit_3 = (R_Digit_4-R_Digit_3)/(Divider/100);
Digit_3 = uint8(Q_Digit_3);
%Digit_3 done

R_Digit_2 = rem(R_Digit_3,Divider/1000);
Q_Digit_2 = (R_Digit_3-R_Digit_2)/(Divider/1000);
Digit_2 = uint8(Q_Digit_2);
%Digit_2 done

R_Digit_1 = rem(R_Digit_2,Divider/10000);
Q_Digit_1 = (R_Digit_2-R_Digit_1)/(Divider/10000);
Digit_1 = uint8(Q_Digit_1);
%Digit_1 done
end

== stateflow chart C28069_LLC_ePWM_V8_230307_PhaeShiftWorking/CloseLoop & Update @ ADCINT, 50kHz/Close Loop Regulation2/If Action Subsystem/Chart3 ==
  note: [output_freq>180]
      | {
      | output_freq=180;
      | output_deadband =  output_deadband + 1;
      | }
  (default) -> (junction 221)
  (junction 221) -> (junction 223) : {
      | %%y(k) = b0*e(k) + b1*e(k-1) - a1*y(k-1)
      | output_freq = (b0*error) + (b1*error_z1) - (a1*output_z1);
      | }
  (junction 223) -> (junction 239) [order 2] : [output_freq<0.65]
  (junction 223) -> (junction 243) [order 3]
  (junction 239) -> (junction 241) : {output_freq=0.65;}
  (junction 223) -> (junction 225) [order 1] : [output_freq>1.5]
  (junction 243) -> (junction 245)
  (junction 225) -> (junction 237) : {output_freq=1.5;}
  (junction 241) -> (junction 237)
  (junction 245) -> (junction 237)
  (junction 237) -> (junction 233) : {
      | output_z1 = output_freq;
      | error_z1 = error;
      | }
  data: output_freq output double =0; error input double; prev_freq input double; b0 input; b1 input; a1 input; error_z1 local =0; output_z1 local =0

== stateflow chart C28069_LLC_ePWM_V8_230307_PhaeShiftWorking/CloseLoop & Update @ ADCINT, 50kHz/Close Loop Regulation2/If Action Subsystem/Chart4 ==
  note: lower limit cap
  note: upper limit cap
  note: reduce duty cycle
  note: increase duty cycle
  note: If dutycycle hit certain %,
      | we set pwm to 0
  note: set to upper limit
      | if pwm = 0
  (default) -> (junction 221)
  (junction 221) -> (junction 223) : {
      | %%y(k) = b0*e(k) + b1*e(k-1) - a1*y(k-1)
      | output_freq = (b0*error) + (b1*error_z1) - (a1*output_z1);
      | }
  (junction 223) -> (junction 239) [order 2] : [output_freq<0.65]
  (junction 223) -> (junction 243) [order 3]
  (junction 243) -> (junction 267) [order 2]
  (junction 267) -> (junction 272) [order 2]
  (junction 267) -> (junction 273) [order 1] : [output_freq==0]
      | {output_freq=1.5;}
  (junction 239) -> (junction 241) : {output_freq=0.65;}
  (junction 223) -> (junction 225) [order 1] : [output_freq>1.5]
  (junction 243) -> (junction 245) [order 1] : [output_deadband>1]
      | {output_deadband = output_deadband - 1;}
  (junction 272) -> (junction 275)
  (junction 225) -> (junction 249) : {
      | output_freq=1.5;
      | output_deadband = output_deadband +1;
      | }
  (junction 249) -> (junction 257) [order 2]
  (junction 257) -> (junction 250)
  (junction 249) -> (junction 251) [order 1] : [output_deadband > 660]
      | {
      | output_deadband = 660;
      | output_freq=0;
      | }
  (junction 250) -> (junction 251)
  (junction 251) -> (junction 237)
  (junction 275) -> (junction 273)
  (junction 273) -> (junction 245)
  (junction 241) -> (junction 237)
  (junction 245) -> (junction 237)
  (junction 237) -> (junction 233) : {
      | output_z1 = output_freq;
      | error_z1 = error;
      | }
  data: output_freq output double =0; error input double; prev_freq input double; b0 input; b1 input; a1 input; error_z1 local =0; output_z1 local =0; output_deadband output

== stateflow chart C28069_LLC_ePWM_V8_230307_PhaeShiftWorking/GetADC, FaultProtection, SoftStart  @5KHz/UpdatePWM/Close Loop Regulation/If Action Subsystem/Chart ==
  note: Note
      | Voltage drop = Freq increase
  note: When Actual voltage is higher
  note: When Actual voltage is lower
  (default) -> (junction 1)
  (junction 1) -> (junction 16) [order 1] : [input_u>0]{output_y=prev_freq-0.01;}
  (junction 1) -> (junction 17) [order 2] : {output_y=prev_freq+0.01;}
  (junction 16) -> (junction 19) [order 1] : [output_y<100]{output_y=100;}
  (junction 17) -> (junction 19) [order 1] : [output_y>180]{output_y=180;}
  (junction 17) -> (junction 32) [order 2]
  (junction 16) -> (junction 34) [order 2]
  (junction 32) -> (junction 19)
  (junction 34) -> (junction 19)
  (junction 19) -> (junction 22)
  data: output_y output double; input_u input double; prev_freq input double

== stateflow chart C28069_LLC_ePWM_V8_230307_PhaeShiftWorking/GetADC, FaultProtection, SoftStart  @5KHz/SoftStart/If Action Subsystem/ReservseSoftStart/Chart1 ==
  note: Under 5KHz, 1 = 0.0002s/cycle
      | 1000 = 0.2s per increment/decrement
  note: [Frequency_Adjusted == Resonant_Frequency]
      | will go here
  note: To initialise the frequency
  note: For increment of 110 (+-5% each DC)
      | Duty_Adjusted @ 660 = 15% Duty
      | '' @ 770 = 10% Duty
      | - - - - - - - - - - - - - - - -
      | 715 + 55 = 15% DutyCycle
      | 660 + 55 (+-2.5%DC) = ~18% DutyCycle = 1us (Minimum required)
  (default) -> (junction 47)
  (junction 47) -> (junction 62) [order 2]
  (junction 62) -> (junction 64) : {
      | First_Pass = 1;
      | Soft_Start = 1;
      | Local_counter = 1;
      | SoftStart_OK = 0;
      | Duty_Adjusted = 100;
      | }
  (junction 47) -> (junction 48) [order 1] : [PFC_OK]
  (junction 48) -> (junction 49) [order 1] : [First_Pass]
  (junction 48) -> (junction 56) [order 2] : [Soft_Start]
  (junction 56) -> (junction 58) [order 1] : [Local_counter > 600]
      | {
      | Local_counter = 0;
      | }
  (junction 58) -> (junction 74) [order 2]
  (junction 74) -> (junction 81) [order 1] : [abs(Frequency_Adjusted - Resonant_Frequency)<1]
  (junction 48) -> (junction 105) [order 4]
  (junction 49) -> (junction 60) : {
      | Frequency_Adjusted = Initial_Frequency;
      | First_Pass = 0;
      | }
  (junction 48) -> (junction 102) [order 3] : [Duty_Adjusted <= 550]
  (junction 56) -> (junction 70) [order 2] : {
      | Local_counter = Local_counter +1;
      | }
  (junction 58) -> (junction 68) [order 1] : [Frequency_Adjusted > Resonant_Frequency]
      | {
      | Frequency_Adjusted = Frequency_Adjusted - 0.1;
      | }
  (junction 74) -> (junction 76) [order 2] : [Frequency_Adjusted < Resonant_Frequency]
      |
      | {
      | Frequency_Adjusted = Frequency_Adjusted + 0.1;
      | }
  (junction 81) -> (junction 84) : {
      | SoftStart_OK = 1;
      | Soft_Start = 0;
      | %%Frequency_Adjusted = Initial_Frequency;
      | }
  (junction 102) -> (junction 105) [order 2] : {
      | Local_counter = Local_counter +1;
      | }
  (junction 105) -> (junction 51)
  (junction 102) -> (junction 108) [order 1] : [Local_counter >600]
      | {
      | Local_counter = 0;
      | }
  (junction 108) -> (junction 51) : {
      | Duty_Adjusted = Duty_Adjusted + 55;
      | }
  (junction 64) -> (junction 60)
  (junction 60) -> (junction 51)
  (junction 51) -> (junction 70)
  (junction 70) -> (junction 68)
  (junction 68) -> (junction 76)
  (junction 84) -> (junction 76)
  data: SoftStart_OK output; Duty_Adjusted output =100; PFC_OK input; Initial_Frequency input; Resonant_Frequency input; Local_counter local =1; Frequency_Adjusted output double; First_Pass local =1; Soft_Start local =1

== stateflow chart C28069_LLC_ePWM_V8_230307_PhaeShiftWorking/GetADC, FaultProtection, SoftStart  @5KHz/SoftStart/If Action Subsystem/SoftStart/Chart1 ==
  note: Under 5KHz, 1 = 0.0002s/cycle
      | 1000 = 0.2s per increment/decrement
  note: [Frequency_Adjusted == Resonant_Frequency]
      | will go here
  note: To initialise the frequency
  (default) -> (junction 47)
  (junction 47) -> (junction 62) [order 2]
  (junction 62) -> (junction 64) : {
      | First_Pass = 1;
      | Soft_Start = 1;
      | Local_counter = 1;
      | SoftStart_OK = 0;
      | }
  (junction 47) -> (junction 48) [order 1] : [PFC_OK]
  (junction 48) -> (junction 49) [order 1] : [First_Pass]
  (junction 48) -> (junction 56) [order 2] : [Soft_Start]
  (junction 56) -> (junction 58) [order 1] : [Local_counter > 400]
      | {
      | Local_counter = 0;
      | }
  (junction 58) -> (junction 74) [order 2]
  (junction 74) -> (junction 81) [order 1] : [[abs(Frequency_Adjusted - Resonant_Frequency)<1]]
  (junction 49) -> (junction 60) : {
      | Frequency_Adjusted = Initial_Frequency;
      | First_Pass = 0;
      | }
  (junction 48) -> (junction 51) [order 3]
  (junction 56) -> (junction 70) [order 2] : {
      | Local_counter = Local_counter +1;
      | }
  (junction 58) -> (junction 68) [order 1] : [Frequency_Adjusted > Resonant_Frequency]
      | {
      | Frequency_Adjusted = Frequency_Adjusted - 0.1;
      | }
  (junction 74) -> (junction 76) [order 2] : [Frequency_Adjusted < Resonant_Frequency]
      |
      | {
      | Frequency_Adjusted = Frequency_Adjusted + 0.1;
      | }
  (junction 81) -> (junction 84) : {
      | SoftStart_OK = 1;
      | Soft_Start = 0;
      | %Frequency_Adjusted = Initial_Frequency;
      | }
  (junction 64) -> (junction 60)
  (junction 60) -> (junction 51)
  (junction 51) -> (junction 70)
  (junction 70) -> (junction 68)
  (junction 68) -> (junction 76)
  (junction 84) -> (junction 76)
  data: SoftStart_OK output; PFC_OK input; Initial_Frequency input; Resonant_Frequency input; Local_counter local =1; Frequency_Adjusted output; First_Pass local =1; Soft_Start local =1

== stateflow chart C28069_LLC_ePWM_V8_230307_PhaeShiftWorking/CloseLoop & Update @ ADCINT, 50kHz/Close Loop Regulation2/If Action Subsystem/Chart6 ==
  note: TBPRD Lower Limit
      | (Highest Frequency)
  note: TBPRD Upper Limit
      | (Lowest Frequency)
  note: [output_freq>180]
      | {
      | output_freq=180;
      | output_deadband =  output_deadband + 1;
      | }
  (default) -> (junction 221)
  (junction 221) -> (junction 223) : {
      | %%y(k) = b0*e(k) + b1*e(k-1) - a1*y(k-1)
      | output_freq = (b0*error) + (b1*error_z1) - (a1*output_z1);
      | }
  (junction 223) -> (junction 239) [order 2] : [output_freq<0.77]
  (junction 223) -> (junction 243) [order 3]
  (junction 243) -> (junction 281) [order 2]
  (junction 281) -> (junction 286)
  (junction 239) -> (junction 294) : {
      | output_freq=0.77;
      | PhaseShift = PhaseShift + 1;
      | }
  (junction 223) -> (junction 225) [order 1] : [output_freq>1.79]
  (junction 243) -> (junction 245) [order 1] : [PhaseShift > 0]
      |
      | {
      | PhaseShift = PhaseShift - 1;
      | }
  (junction 281) -> (junction 283) [commented out] : [output_freq == 0]
      |
      | {
      | output_freq = 1.79;
      | }
  (junction 286) -> (junction 288)
  (junction 225) -> (junction 237) : {
      | output_freq=1.79;
      | }
  (junction 294) -> (junction 300) [order 2]
  (junction 294) -> (junction 292) [order 1] : [PhaseShift > 150]
      | {
      | PhaseShift = 150;
      | %output_freq=0;
      | }
  (junction 300) -> (junction 302)
  (junction 302) -> (junction 292)
  (junction 292) -> (junction 241)
  (junction 241) -> (junction 237)
  (junction 245) -> (junction 237)
  (junction 283) -> (junction 245)
  (junction 288) -> (junction 283)
  (junction 237) -> (junction 233) : {
      | output_z1 = output_freq;
      | error_z1 = error;
      | }
  (junction 233) -> (junction 249) : %%{output_freq=1;}
  data: output_freq output double =0; error input double; prev_freq input double; b0 input; b1 input; a1 input; error_z1 local =0; output_z1 local =0; PhaseShift output double =0
